simulink model "SimForcesGP2020a"  (R2020b)
settings: Solver=ode4  StartTime=0.0  StopTime=10  FixedStep=0.001  MaxStep=0.001  RelTol=1e-7
values from neighbouring files (symbols this model uses):
  B11_r_B11C = [0.23805608; 0.13201777; 0]    [InitializeSimulationGP.m]
  B11_r_B11Tc1 = [L11; 0; 0]    [InitializeSimulationGP.m]
  B11_Rot_Tc1 = eye(3)    [InitializeSimulationGP.m]
  B11cI = [0.28426000 -0.06487287 0;         -0.06487287  0.54237481 0;                   0  0          0.67891020]    [InitializeSimulationGP.m]
  B12_r_B12C = [0.60504569; 0.27199376; 0.00002484]    [InitializeSimulationGP.m]
  B12_r_B12Tc2 = [L21;0;0]    [InitializeSimulationGP.m]
  B12_Rot_Tc2 = eye(3)    [InitializeSimulationGP.m]
  B12cI = [1.18803886 -2.36786418 0.00280315;          -2.36786418 6.31493281 0.00022322;           0.00280315 0.00022322 7.40915161]    [InitializeSimulationGP.m]
  B31_r_B31C = [0.35781210 0 0]    [InitializeSimulationGP.m]
  B31_Rot_B41 = eye(3)    [InitializeSimulationGP.m]
  B31cI = diag([0.03150902 0.90735702 0.90763033])    [InitializeSimulationGP.m]
  B32_r_B32C = [0.35781210 0 0]    [InitializeSimulationGP.m]
  B32_Rot_B42 = eye(3)    [InitializeSimulationGP.m]
  B32cI = diag([0.03150902 0.90735702 0.90763033])    [InitializeSimulationGP.m]
  B41_r_B41C = [0.55785997 0 0]    [InitializeSimulationGP.m]
  B41_r_B41Tc1 = [lc1;0;0]    [InitializeSimulationGP.m]
  B41cI = diag([0.00370720 0.55759812 0.55785997])    [InitializeSimulationGP.m]
  B42_r_B42C = [0.55785997 0 0]    [InitializeSimulationGP.m]
  B42_r_B42Tc2 = [lc2; 0; 0]    [InitializeSimulationGP.m]
  B42cI = diag([0.00370720 0.55759812 0.55785997])    [InitializeSimulationGP.m]
  B52_r_B52C = [0 0 0.56802906]    [InitializeSimulationGP.m]
  B52_r_B52P32 = [lc3; 0; 0]    [InitializeSimulationGP.m]
  B52_Rot_P32 = eye(3)    [InitializeSimulationGP.m]
  B52cI = diag([0.91789884, 0.91790043, 0.00091463])    [InitializeSimulationGP.m]
  Bc1_r_Bc1B11 = [L1; 0; 0]    [InitializeSimulationGP.m]
  Bc1_r_Bc1B31 = [0;0;0]    [InitializeSimulationGP.m]
  Bc1_r_Bc1C = [0.14178771; 0.16555780; 0]    [InitializeSimulationGP.m]
  Bc1_V = [0;0;0;0;0;0]    [InitializeSimulationGP.m]
  Bc1cI = [+5.892211080 +5.476111360 -0.000019630;          +5.476111360 +28.66965601 -0.000024550;          -0.000019630 -0.000024550 +29.78955950]    [InitializeSimulationGP.m]
  Bc2_r_Bc2B12 = [L2;0;0]    [InitializeSimulationGP.m]
  Bc2_r_Bc2B32 = [0;0;0]    [InitializeSimulationGP.m]
  Bc2_r_Bc2C = [0.54319901; 0.10543875; 0]    [InitializeSimulationGP.m]
  Bc2cI = [0.48071390 0.52924041 0;          0.52924041 5.80912352 0;              0      0          5.97255351]    [InitializeSimulationGP.m]
  beta1 = atan2d(374.261,935)*pi/180    [InitializeSimulationGP.m]
  beta2 = atan2d(45.757,373.313)*pi/180    [InitializeSimulationGP.m]
  beta3 = atan2d(139.50,1132.19)*pi/180    [InitializeSimulationGP.m]
  beta4 = atan2d(88.061,296.198)*pi/180    [InitializeSimulationGP.m]
  D22F = [0;0;0;0;0;0]    [InitializeSimulationGP.m]
  L1 = 1.0071227324212    (= 1.00712273242)    [InitializeSimulationGP.m]
  L11 = 0.37610632101293    (= 0.376106321013)    [InitializeSimulationGP.m]
  L2 = 1.132185817991    (= 1.13218581799)    [InitializeSimulationGP.m]
  L21 = 0.30901132665325    (= 0.309011326653)    [InitializeSimulationGP.m]
  lc1 = 0.745    [InitializeSimulationGP.m]
  lc2 = 0.745    [InitializeSimulationGP.m]
  mB11 = 25.52660174    [InitializeSimulationGP.m]
  mB12 = 33.92850233    [InitializeSimulationGP.m]
  mB31 = 17.36281648    [InitializeSimulationGP.m]
  mB32 = 17.36281648    [InitializeSimulationGP.m]
  mB41 = 10.34519231    [InitializeSimulationGP.m]
  mB42 = 10.34519231    [InitializeSimulationGP.m]
  mB52 = 6.73059863    [InitializeSimulationGP.m]
  mBc1 = 307.29601379    [InitializeSimulationGP.m]
  mBc2 = 54.58702836    [InitializeSimulationGP.m]
  mP22 = 9.26136143    [InitializeSimulationGP.m]
  mP32 = 570.18877059    [InitializeSimulationGP.m]
  P22_r_P22C = [0.62192523 0 0]    [InitializeSimulationGP.m]
  P22_Rot_B52 = eye(3)    [InitializeSimulationGP.m]
  P22cI = diag([0.00662754, 1.48387017, 1.48398069])    [InitializeSimulationGP.m]
  P32_r_P32C = [0.25466704; -0.13034397; -0.01302248]    [InitializeSimulationGP.m]
  P32_r_P32D22 = [0.40499744871392; -0.13130517281345; -0.013385243295654]    [InitializeSimulationGP.m]
  P32_Rot_D22 = [1 0 0;              0 0.9707729441837 0.23999977258512;              0 -0.23999977258512 0.9707729441837]    [InitializeSimulationGP.m]
  P32cI = [46.81220713 0.38607676 -0.00453819;          0.38607676 71.92201786 -1.14320993;          -0.00453819 -1.14320993 67.38128576]    [InitializeSimulationGP.m]
  Tc1_r_Tc1Bc2 = [0.098495302558553; 0.01838181329939; 0]    [InitializeSimulationGP.m]
  Tc1_Rot_Bc2 = [cos(alpha2) -sin(alpha2) 0;                sin(alpha2)  cos(alpha2) 0;                0            0           1]    [InitializeSimulationGP.m]
  Tc2_r_Tc2P22 = [-0.048858374920227;0.36587359346146;0.035276938723102]    [InitializeSimulationGP.m]
  Tc2_Rot_P22 = [0.95853460763586 -0.27664713597974  0.0683942111482;                0.28497614981675  0.93051946315663 -0.23004808784757;                0                 0.23999977258511  0.9707729441837]    [InitializeSimulationGP.m]
  Th1A = 5*pi/180    (= 0.0872664625997)    [InitializeSimulationGP.m]
  Th1B = 20*pi/180    (= 0.349065850399)    [InitializeSimulationGP.m]
  Th1f = 1    [InitializeSimulationGP.m]
  Th2A = 15*pi/180    (= 0.261799387799)    [InitializeSimulationGP.m]
  Th2B = -50*pi/180    (= -0.872664625997)    [InitializeSimulationGP.m]
  Th2f = 2    [InitializeSimulationGP.m]
  W_r_WBc1 = [0.185;-0.085;0]    [InitializeSimulationGP.m]
  W_Rot_Bc1 = [cos(alpha1) -sin(alpha1) 0;              sin(alpha1)  cos(alpha1) 0;              0            0           1]    [InitializeSimulationGP.m]
  Wg = [0; 9.8066; 0]    [InitializeSimulationGP.m]
  x10 = 0.83    [InitializeSimulationGP.m]
  x20 = 0.83    [InitializeSimulationGP.m]
  xf = [1;0;0;0;0;0]    [InitializeSimulationGP.m]
  xt2A = 0.1    [InitializeSimulationGP.m]
  xt2B = 0.5    [InitializeSimulationGP.m]
  xt2f = 1    [InitializeSimulationGP.m]
  ztau = [0;0;0;0;0;1]    [InitializeSimulationGP.m]
undefined symbols (not defined in the file or in its folder): B11_V, B11_V_SS, B11Ftot, B12_U_Tc2, B12_V, B12_V_SS, B12Ftot, B31_r_B31B41, B31_V, B31_V_SS, B31FTot, B32_r_B32B42, B32_U_B42, B32_V, B32_V_SS, B32FTot, B41_V, B41_V_SS, B41FTot, B42_Rot_Tc2, B42_U_Tc2, B42_V, B42_V_SS, B42FTot, B52_U_P32, B52_V, B52_V_SS, B52Ftot, Bc1_V_SS, Bc1Tot, Bc2_Rot_B12, Bc2_Rot_B32, Bc2_U_B12, Bc2_U_B32, Bc2_V, Bc2_V_SS, Bc2Tot, D22_V, D22_V_SS, dq1, dq11, dq12, dq2, dq21, dq22, dx1, dx2, FTot_S1, FTot_S2P, FTot_S2R, P22_r_P22B52, P22_U_B52, P22_V, P22_V_SS, P22FTot, P32_U_D22, P32_V, P32_V_SS, P32FTot, q1 ... (+28)
libraries: nesl_utility x94, sm_lib x45
(part 5 of 6)

== system SimForcesGP2020a/Hydraulic manipulator, calculation/AnalyticVelocities/Structure 2 (Revolute segment)/GeomPropS2R/TiltPistonVelocity ==
  note: Pass to output...
  note: Process data...
  note: Get inputs...
  dq2 : Inport
  x2 : Inport  Port=2
  q2 : Inport  Port=3
  TiltPistonVelocity : MATLAB Function  TreatAsAtomicUnit=on
  dx2 : Outport
  wires:
  dq2/1 -> [dq2]  "dq2"
  [dq2] -> TiltPistonVelocity/3(dq2)  "dq2"
  x2/1 -> [x2]  "x2"
  [x2] -> TiltPistonVelocity/1(x2)  "x2"
  q2/1 -> [q2]  "q2"
  [q2] -> TiltPistonVelocity/2(q2)  "q2"
  [dx2] -> dx2/1  "dx2"
  TiltPistonVelocity/1(dx2) -> [dx2]  "dx2"

== system SimForcesGP2020a/Hydraulic manipulator, calculation/AnalyticVelocities/Structure 2 (Revolute segment)/GeomPropS2R/q21-angle ==
  note: Pass to outputs...
  note: Process data...
  note: Get inputs...
  x2 : Inport
  Fcn : Fcn  Expr=-acos((L21*L21-(u+x20)*(u+x20)-L2*L2)/(-2*(u+x20)*L2))
  q21 : Outport
  wires:
  x2/1 -> [x2]
  [q21] -> q21/1
  [x2] -> Fcn/1
  Fcn/1 -> [q21]

== system SimForcesGP2020a/Hydraulic manipulator, calculation/AnalyticVelocities/Structure 2 (Revolute segment)/GeomPropS2R/q22-angle ==
  note: Get inputs...
  note: Process data...
  note: Pass to outputs...
  x2 : Inport
  Fcn : Fcn  Expr=-acos((L2*L2-(u+x20)*(u+x20)-L21*L21)/(-2*(u+x20)*L21))
  q22 : Outport
  wires:
  [q22] -> q22/1
  Fcn/1 -> [q22]
  [x2] -> Fcn/1
  x2/1 -> [x2]

== system SimForcesGP2020a/Hydraulic manipulator, calculation/AnalyticVelocities/Structure 2 (Revolute segment)/GeomPropS2R/q2Derivative ==
  note: Pass to outputs...
  note: Process data...
  note: Get inputs...
  q2 : Inport
  Derivative4 : Derivative
  dq2 : Outport
  wires:
  q2/1 -> [q2]  "q2"
  [q2] -> Derivative4/1  "q2"
  [dq2] -> dq2/1  "dq2"
  Derivative4/1 -> [dq2]  "dq2"

== matlab function SimForcesGP2020a/Hydraulic manipulator, calculation/AnalyticVelocities/Structure 1/UMatsS1/B41_U_Tc1 ==
  data: B41_r_B41Tc1 input; B41_U_Tc1 output; B41_Rot_Tc1 input
function B41_U_Tc1 = B41_U_Tc1(B41_r_B41Tc1, B41_Rot_Tc1)

B41_U_Tc1 = [B41_Rot_Tc1,                    zeros(3);...
             dual(B41_r_B41Tc1)*B41_Rot_Tc1, B41_Rot_Tc1];
   
end
   
function dual_r = dual(ArAB)

dual_r = [0,  -ArAB(3), ArAB(2);...
          ArAB(3), 0, -ArAB(1);...
          -ArAB(2), ArAB(1), 0];

end

== matlab function SimForcesGP2020a/Hydraulic manipulator, calculation/AnalyticVelocities/Structure 1/RotMatsS1/B41_Rot_Tc1 ==
  data: q12 input; B41_Rot_Tc1 output
function B41_Rot_Tc1 = B41_Rot_Tc1(q12)

B41_Rot_Tc1 = [+cos(q12) -sin(q12) 0;...
               +sin(q12) +cos(q12) 0;...
                   0        0      1];

== matlab function SimForcesGP2020a/Hydraulic manipulator, calculation/AnalyticVelocities/Structure 2 (Prismatic segment)/PosVecsS2P/P22_r_P22B52 ==
  data: xt2 input; P22_r_P22B52 output; P22_r_P22P22p parameter
function P22_r_P22B52 = P22_r_P22B52(xt2, P22_r_P22P22p)

% position vector of {B41} frame at lift piston tip w.r.t. {B31} frame at 
% lift cylinder connection point [m]
P22_r_P22B52 = P22_r_P22P22p + [xt2; 0; 0];

== matlab function SimForcesGP2020a/Hydraulic manipulator, calculation/AnalyticVelocities/Structure 1/UMatsS1/Bc1_U_B11 ==
  data: Bc1_r_Bc1B11 input; Bc1_U_B11 output; Bc1_Rot_B11 input
function Bc1_U_B11 = Bc1_U_B11(Bc1_r_Bc1B11, Bc1_Rot_B11)

Bc1_U_B11 = [Bc1_Rot_B11,                    zeros(3);...
             dual(Bc1_r_Bc1B11)*Bc1_Rot_B11, Bc1_Rot_B11];
   
end
   
function dual_r = dual(ArAB)

dual_r = [0,  -ArAB(3), ArAB(2);...
          ArAB(3), 0, -ArAB(1);...
          -ArAB(2), ArAB(1), 0];

end

== matlab function SimForcesGP2020a/Hydraulic manipulator, calculation/AnalyticVelocities/Structure 2 (Prismatic segment)/UMatsS2P/P22_U_B52 ==
  data: P22_r_P22B52 input; P22_U_B52 output; P22_Rot_B52 input
function P22_U_B52 = P22_U_B52(P22_r_P22B52, P22_Rot_B52)

P22_U_B52 = [P22_Rot_B52,                    zeros(3);...
             dual(P22_r_P22B52)*P22_Rot_B52, P22_Rot_B52];
   
end
   
function dual_r = dual(ArAB)

dual_r = [0,  -ArAB(3), ArAB(2);...
          ArAB(3), 0, -ArAB(1);...
          -ArAB(2), ArAB(1), 0];

end

== matlab function SimForcesGP2020a/Hydraulic manipulator, calculation/AnalyticVelocities/Structure 2 (Prismatic segment)/UMatsS2P/B52_U_P32 ==
  data: B52_r_B52B32 input; B52_U_P32 output; B52_Rot_B32 input
function B52_U_P32 = B52_U_P32(B52_r_B52B32, B52_Rot_B32)

B52_U_P32 = [B52_Rot_B32,                    zeros(3);...
             dual(B52_r_B52B32)*B52_Rot_B32, B52_Rot_B32];
   
end
   
function dual_r = dual(ArAB)

dual_r = [0,  -ArAB(3), ArAB(2);...
          ArAB(3), 0, -ArAB(1);...
          -ArAB(2), ArAB(1), 0];

end

== matlab function SimForcesGP2020a/Hydraulic manipulator, calculation/AnalyticVelocities/Structure 2 (Revolute segment)/PosVecsS2R/B32_r_B32B42 ==
  data: x2 input; B32_r_B32B42 output; B32_r_B32B32p parameter
function B32_r_B32B42 = B32_r_B32B42(x2, B32_r_B32B32p)

B32_r_B32B42 = B32_r_B32B32p + [x2;0;0];

== matlab function SimForcesGP2020a/Hydraulic manipulator, calculation/AnalyticVelocities/Structure 2 (Revolute segment)/RotMatsS2R/B42_Rot_Tc2 ==
  data: q22 input; B42_Rot_Tc2 output
function B42_Rot_Tc2 = B42_Rot_Tc2(q22)

B42_Rot_Tc2 = [+cos(q22) -sin(q22) 0;...
               +sin(q22) +cos(q22) 0;...
                   0        0      1];

== matlab function SimForcesGP2020a/Hydraulic manipulator, calculation/AnalyticVelocities/Structure 2 (Revolute segment)/RotMatsS2R/Bc2_Rot_B12 ==
  data: q2 input; Bc2_Rot_B12 output
function Bc2_Rot_B12 = Bc2_Rot_B12(q2)

Bc2_Rot_B12 = [+cos(q2) -sin(q2) 0;...
               +sin(q2) +cos(q2) 0;...
                  0        0     1];

== matlab function SimForcesGP2020a/Hydraulic manipulator, calculation/AnalyticVelocities/Structure 2 (Revolute segment)/RotMatsS2R/Bc2_Rot_B32 ==
  data: q21 input; Bc2_Rot_B32 output

function Bc2_Rot_B32 = Bc2_Rot_B32(q21)

Bc2_Rot_B32 = [+cos(q21) -sin(q21) 0;...
               +sin(q21) +cos(q21) 0;...
                   0         0     1];

== matlab function SimForcesGP2020a/Hydraulic manipulator, calculation/AnalyticVelocities/Structure 2 (Revolute segment)/UMatS2R/B12_U_Tc2 ==
  data: B12_r_B12Tc2 input; B12_U_Tc2 output; B12_Rot_Tc2 input
function B12_U_Tc2 = B12_U_Tc2(B12_r_B12Tc2, B12_Rot_Tc2)

B12_U_Tc2 = [B12_Rot_Tc2,                    zeros(3);...
             dual(B12_r_B12Tc2)*B12_Rot_Tc2, B12_Rot_Tc2];
   
end
   
function dual_r = dual(ArAB)

dual_r = [0,  -ArAB(3), ArAB(2);...
          ArAB(3), 0, -ArAB(1);...
          -ArAB(2), ArAB(1), 0];

end

== matlab function SimForcesGP2020a/Hydraulic manipulator, calculation/AnalyticVelocities/Structure 2 (Revolute segment)/UMatS2R/B32_U_B42 ==
  data: B32_r_B32B42 input; B32_U_B42 output; B32_Rot_B42 input
function B32_U_B42 = B32_U_B42(B32_r_B32B42, B32_Rot_B42)

B32_U_B42 = [B32_Rot_B42,                    zeros(3);...
             dual(B32_r_B32B42)*B32_Rot_B42, B32_Rot_B42];
   
end
   
function dual_r = dual(ArAB)

dual_r = [0,  -ArAB(3), ArAB(2);...
          ArAB(3), 0, -ArAB(1);...
          -ArAB(2), ArAB(1), 0];

end

== matlab function SimForcesGP2020a/Hydraulic manipulator, calculation/AnalyticVelocities/Structure 2 (Revolute segment)/UMatS2R/B42_U_Tc2 ==
  data: B42_r_B42Tc2 input; B42_U_Tc2 output; B42_Rot_Tc2 input
function B42_U_Tc2 = B42_U_Tc2(B42_r_B42Tc2, B42_Rot_Tc2)

B42_U_Tc2 = [B42_Rot_Tc2,                    zeros(3);...
             dual(B42_r_B42Tc2)*B42_Rot_Tc2, B42_Rot_Tc2];
   
end
   
function dual_r = dual(ArAB)

dual_r = [0,  -ArAB(3), ArAB(2);...
          ArAB(3), 0, -ArAB(1);...
          -ArAB(2), ArAB(1), 0];

end

== matlab function SimForcesGP2020a/Hydraulic manipulator, calculation/AnalyticVelocities/Structure 2 (Revolute segment)/UMatS2R/Bc2_U_B12 ==
  data: Bc2_r_Bc2B12 input; Bc2_U_B12 output; Bc2_Rot_B12 input
function Bc2_U_B12 = Bc2_U_B12(Bc2_r_Bc2B12, Bc2_Rot_B12)

Bc2_U_B12 = [Bc2_Rot_B12,                    zeros(3);...
             dual(Bc2_r_Bc2B12)*Bc2_Rot_B12, Bc2_Rot_B12];
   
end
   
function dual_r = dual(ArAB)

dual_r = [0,  -ArAB(3), ArAB(2);...
          ArAB(3), 0, -ArAB(1);...
          -ArAB(2), ArAB(1), 0];

end

== matlab function SimForcesGP2020a/Hydraulic manipulator, calculation/AnalyticVelocities/Structure 1/RotMatsS1/Bc1_Rot_B11 ==
  data: q1 input; Bc1_Rot_B11 output
function Bc1_Rot_B11 = Bc1_Rot_B11(q1)

Bc1_Rot_B11 = [+cos(q1) -sin(q1) 0;...
               +sin(q1) +cos(q1) 0;...
                  0        0     1];

== matlab function SimForcesGP2020a/Hydraulic manipulator, calculation/AnalyticVelocities/Structure 2 (Revolute segment)/UMatS2R/Bc2_U_B32 ==
  data: Bc2_r_Bc2B32 input; Bc2_U_B32 output; Bc2_Rot_B32 input
function Bc2_U_B32 = Bc2_U_B32(Bc2_r_Bc2B32, Bc2_Rot_B32)

Bc2_U_B32 = [Bc2_Rot_B32,                    zeros(3);...
             dual(Bc2_r_Bc2B32)*Bc2_Rot_B32, Bc2_Rot_B32];
   
end
   
function dual_r = dual(ArAB)

dual_r = [0,  -ArAB(3), ArAB(2);...
          ArAB(3), 0, -ArAB(1);...
          -ArAB(2), ArAB(1), 0];

end

== matlab function SimForcesGP2020a/Hydraulic manipulator, calculation/AnalyticVelocities/Structure 1/UMatsS1/Tc1_U_Bc2 ==
  data: Tc1_r_Tc1Bc2 input; Tc1_U_Bc2 output; Tc1_Rot_Bc2 input
function Tc1_U_Bc2 = Tc1_U_Bc2(Tc1_r_Tc1Bc2, Tc1_Rot_Bc2)

Tc1_U_Bc2 = [Tc1_Rot_Bc2,                    zeros(3);...
             dual(Tc1_r_Tc1Bc2)*Tc1_Rot_Bc2, Tc1_Rot_Bc2];
   
end
   
function dual_r = dual(ArAB)

dual_r = [0,  -ArAB(3), ArAB(2);...
          ArAB(3), 0, -ArAB(1);...
          -ArAB(2), ArAB(1), 0];

end

== matlab function SimForcesGP2020a/Hydraulic manipulator, calculation/AnalyticVelocities/Structure 2 (Revolute segment)/UMatS2R/Tc2_U_P22 ==
  data: Tc2_r_Tc2P22 input; Tc2_U_P22 output; Tc2_Rot_P22 input
function Tc2_U_P22 = Tc2_U_P22(Tc2_r_Tc2P22, Tc2_Rot_P22)

Tc2_U_P22 = [Tc2_Rot_P22,                    zeros(3);...
             dual(Tc2_r_Tc2P22)*Tc2_Rot_P22, Tc2_Rot_P22];
   
end
   
function dual_r = dual(ArAB)

dual_r = [0,  -ArAB(3), ArAB(2);...
          ArAB(3), 0, -ArAB(1);...
          -ArAB(2), ArAB(1), 0];

end

== matlab function SimForcesGP2020a/Hydraulic manipulator, calculation/AnalyticTotalForces/Structure 1/MATLAB Function2 ==
  data: thetaB11 output; B11_r_B11C parameter; mB11 parameter; B11cI parameter
function thetaB11 = thetaB11(B11_r_B11C, mB11, B11cI)

rx = B11_r_B11C(1);
ry = B11_r_B11C(2);
rz = B11_r_B11C(3);

Ixx = B11cI(1,1);
Iyy = B11cI(2,2);
Izz = B11cI(3,3);
Iyz = B11cI(2,3);
Ixz = B11cI(1,3);
Ixy = B11cI(1,2);

t1 = rx*rx;
t2 = ry*ry;
t3 = rz*rz;
t4 = rx*mB11;

thetaB11 = [mB11; rx*mB11; ry*mB11; rz*mB11; t1*mB11; t2*mB11; t3*mB11; t4*ry - Ixy; t4*rz - Ixz; mB11*ry*rz - Iyz; Ixx; Iyy; Izz];

== matlab function SimForcesGP2020a/Hydraulic manipulator, calculation/AnalyticTotalForces/Structure 1/MATLAB Function3 ==
  data: B11V input; B11a input; B11w input; B11dw input; B11_Rot_W input; Wg parameter; YB11 output
function YB11  = thetaBc1(B11V, B11a, B11w, B11dw, B11_Rot_W,  Wg)

vx = B11V(1);
vy = B11V(2);
vz = B11V(3);
ax = B11a(1);
ay = B11a(2);
az = B11a(3);
wx = B11w(1);
wy = B11w(2);
wz = B11w(3);
dwx = B11dw(1);
dwy = B11dw(2);
dwz = B11dw(3);
Bc1g = B11_Rot_W*Wg;
gx = Bc1g(1);
gy = Bc1g(2);
gz = Bc1g(3);

Y11 = ( ax + vz * wy - vy * wz  + gx);
t5 = (wy *  wy);
t6 = (wz * wz);
Y12 = -t5 - t6;
t7 = (wx * wy);
Y13 = (t7 - dwz);
t8 = (wx * wz);
Y14 = (t8 + dwy);
Y15 = 0;
Y16 = 0;
Y17 = 0;
Y18 = 0;
Y19 = 0;
Y110 = 0;
Y111 = 0;
Y112 = 0;
Y113 = 0;
Y21 = vx * wz - vz * wx + ay + gy;
Y22 = t7 + dwz;
t11 = wx * wx;
Y23 = -t11 - t6;
t12 = wy * wz;
Y24 = t12 - dwx;
Y25 = 0;
Y26 = 0;
Y27 = 0;
Y28 = 0;
Y29 = 0;
Y210 = 0;
Y211 = 0;
Y212 = 0;
Y213 = 0;
Y31 = -vx * wy + vy * wx + az + gz;
Y32 = t8 - dwy;
Y33 = t12 + dwx;
Y34 = -t11 - t5;
Y35 = 0;
Y36 = 0;
Y37 = 0;
Y38 = 0;
Y39 = 0;
Y310 = 0;
Y311 = 0;
Y312 = 0;
Y313 = 0;
Y41 = 0;
Y42 = 0;
Y43 = Y31;
Y44 = -Y21;
Y45 = 0;
Y46 = Y33;
Y47 = -Y24;
Y48 = Y32;
Y49 = -Y22;
Y410 = -t5 + t6;
Y411 = dwx;
Y412 = -t12;
Y413 = t12;
Y51 = 0;
Y52 = -Y31;
Y53 = 0;
Y54 = Y11;
Y55 = -Y32;
Y56 = 0;
Y57 = Y14;
Y58 = -Y33;
Y59 = t11 - t6;
Y510 = Y13;
Y511 = t8;
Y512 = dwy;
Y513 = -t8;
Y61 = 0;
Y62 = Y21;
Y63 = -Y11;
Y64 = 0;
Y65 = Y22;
Y66 = -Y13;
Y67 = 0;
Y68 = t5 - t11;
Y69 = Y24;
Y610 = -Y14;
Y611 = -t7;
Y612 = t7;
Y613 = dwz;

YB11 = [Y11 Y12 Y13 Y14 Y15 Y16 Y17 Y18 Y19 Y110 Y111 Y112 Y113;...
        Y21 Y22 Y23 Y24 Y25 Y26 Y27 Y28 Y29 Y210 Y211 Y212 Y213;...
        Y31 Y32 Y33 Y34 Y35 Y36 Y37 Y38 Y39 Y310 Y311 Y312 Y313;...
        Y41 Y42 Y43 Y44 Y45 Y46 Y47 Y48 Y49 Y410 Y411 Y412 Y413;...
        Y51 Y52 Y53 Y54 Y55 Y56 Y57 Y58 Y59 Y510 Y511 Y512 Y513;...
        Y61 Y62 Y63 Y64 Y65 Y66 Y67 Y68 Y69 Y610 Y611 Y612 Y613];

== matlab function SimForcesGP2020a/Hydraulic manipulator, calculation/AnalyticTotalForces/Structure 1/MATLAB Function4 ==
  data: thetaB31 output; B31_r_B31C parameter; mB31 parameter; B31cI parameter
function thetaB31 = thetaB31(B31_r_B31C, mB31, B31cI)

rx = B31_r_B31C(1);
ry = B31_r_B31C(2);
rz = B31_r_B31C(3);

Ixx = B31cI(1,1);
Iyy = B31cI(2,2);
Izz = B31cI(3,3);
Iyz = B31cI(2,3);
Ixz = B31cI(1,3);
Ixy = B31cI(1,2);

t1 = rx*rx;
t2 = ry*ry;
t3 = rz*rz;
t4 = rx*mB31;

thetaB31 = [mB31; rx*mB31; ry*mB31; rz*mB31; t1*mB31; t2*mB31; t3*mB31; t4*ry - Ixy; t4*rz - Ixz; mB31*ry*rz - Iyz; Ixx; Iyy; Izz];

== matlab function SimForcesGP2020a/Hydraulic manipulator, calculation/AnalyticTotalForces/Structure 1/MATLAB Function5 ==
  data: B31V input; B31a input; B31w input; B31dw input; B31_Rot_W input; Wg parameter; YB31 output
function YB31  = thetaBc1(B31V, B31a, B31w, B31dw, B31_Rot_W,  Wg)

vx = B31V(1);
vy = B31V(2);
vz = B31V(3);
ax = B31a(1);
ay = B31a(2);
az = B31a(3);
wx = B31w(1);
wy = B31w(2);
wz = B31w(3);
dwx = B31dw(1);
dwy = B31dw(2);
dwz = B31dw(3);
Bc1g = B31_Rot_W*Wg;
gx = Bc1g(1);
gy = Bc1g(2);
gz = Bc1g(3);

Y11 = ( ax + vz * wy - vy * wz  + gx);
t5 = (wy *  wy);
t6 = (wz * wz);
Y12 = -t5 - t6;
t7 = (wx * wy);
Y13 = (t7 - dwz);
t8 = (wx * wz);
Y14 = (t8 + dwy);
Y15 = 0;
Y16 = 0;
Y17 = 0;
Y18 = 0;
Y19 = 0;
Y110 = 0;
Y111 = 0;
Y112 = 0;
Y113 = 0;
Y21 = vx * wz - vz * wx + ay + gy;
Y22 = t7 + dwz;
t11 = wx * wx;
Y23 = -t11 - t6;
t12 = wy * wz;
Y24 = t12 - dwx;
Y25 = 0;
Y26 = 0;
Y27 = 0;
Y28 = 0;
Y29 = 0;
Y210 = 0;
Y211 = 0;
Y212 = 0;
Y213 = 0;
Y31 = -vx * wy + vy * wx + az + gz;
Y32 = t8 - dwy;
Y33 = t12 + dwx;
Y34 = -t11 - t5;
Y35 = 0;
Y36 = 0;
Y37 = 0;
Y38 = 0;
Y39 = 0;
Y310 = 0;
Y311 = 0;
Y312 = 0;
Y313 = 0;
Y41 = 0;
Y42 = 0;
Y43 = Y31;
Y44 = -Y21;
Y45 = 0;
Y46 = Y33;
Y47 = -Y24;
Y48 = Y32;
Y49 = -Y22;
Y410 = -t5 + t6;
Y411 = dwx;
Y412 = -t12;
Y413 = t12;
Y51 = 0;
Y52 = -Y31;
Y53 = 0;
Y54 = Y11;
Y55 = -Y32;
Y56 = 0;
Y57 = Y14;
Y58 = -Y33;
Y59 = t11 - t6;
Y510 = Y13;
Y511 = t8;
Y512 = dwy;
Y513 = -t8;
Y61 = 0;
Y62 = Y21;
Y63 = -Y11;
Y64 = 0;
Y65 = Y22;
Y66 = -Y13;
Y67 = 0;
Y68 = t5 - t11;
Y69 = Y24;
Y610 = -Y14;
Y611 = -t7;
Y612 = t7;
Y613 = dwz;

YB31 = [Y11 Y12 Y13 Y14 Y15 Y16 Y17 Y18 Y19 Y110 Y111 Y112 Y113;...
        Y21 Y22 Y23 Y24 Y25 Y26 Y27 Y28 Y29 Y210 Y211 Y212 Y213;...
        Y31 Y32 Y33 Y34 Y35 Y36 Y37 Y38 Y39 Y310 Y311 Y312 Y313;...
        Y41 Y42 Y43 Y44 Y45 Y46 Y47 Y48 Y49 Y410 Y411 Y412 Y413;...
        Y51 Y52 Y53 Y54 Y55 Y56 Y57 Y58 Y59 Y510 Y511 Y512 Y513;...
        Y61 Y62 Y63 Y64 Y65 Y66 Y67 Y68 Y69 Y610 Y611 Y612 Y613];

== matlab function SimForcesGP2020a/Hydraulic manipulator, calculation/AnalyticTotalForces/Structure 1/MATLAB Function6 ==
  data: thetaB41 output; B41_r_B41C parameter; mB41 parameter; B41cI parameter
function thetaB41 = thetaB41(B41_r_B41C, mB41, B41cI)

rx = B41_r_B41C(1);
ry = B41_r_B41C(2);
rz = B41_r_B41C(3);

Ixx = B41cI(1,1);
Iyy = B41cI(2,2);
Izz = B41cI(3,3);
Iyz = B41cI(2,3);
Ixz = B41cI(1,3);
Ixy = B41cI(1,2);

t1 = rx*rx;
t2 = ry*ry;
t3 = rz*rz;
t4 = rx*mB41;

thetaB41 = [mB41; rx*mB41; ry*mB41; rz*mB41; t1*mB41; t2*mB41; t3*mB41; t4*ry - Ixy; t4*rz - Ixz; mB41*ry*rz - Iyz; Ixx; Iyy; Izz];

== matlab function SimForcesGP2020a/Hydraulic manipulator, calculation/AnalyticVelocities/Structure 1/UMatsS1/B11_U_Tc1 ==
  data: B11_r_B11Tc1 input; B11_U_Tc1 output; B11_Rot_Tc1 input
function B11_U_Tc1 = B11_U_Tc1(B11_r_B11Tc1, B11_Rot_Tc1)

B11_U_Tc1 = [B11_Rot_Tc1,                    zeros(3);...
             dual(B11_r_B11Tc1)*B11_Rot_Tc1, B11_Rot_Tc1];
   
end
   
function dual_r = dual(ArAB)

dual_r = [0,  -ArAB(3), ArAB(2);...
          ArAB(3), 0, -ArAB(1);...
          -ArAB(2), ArAB(1), 0];

end

== matlab function SimForcesGP2020a/Hydraulic manipulator, calculation/AnalyticTotalForces/Structure 1/MATLAB Function7 ==
  data: B41V input; B41a input; B41w input; B41dw input; B41_Rot_W input; Wg parameter; YB41 output
function YB41  = thetaB41(B41V, B41a, B41w, B41dw, B41_Rot_W,  Wg)

vx = B41V(1);
vy = B41V(2);
vz = B41V(3);
ax = B41a(1);
ay = B41a(2);
az = B41a(3);
wx = B41w(1);
wy = B41w(2);
wz = B41w(3);
dwx = B41dw(1);
dwy = B41dw(2);
dwz = B41dw(3);
Bc1g = B41_Rot_W*Wg;
gx = Bc1g(1);
gy = Bc1g(2);
gz = Bc1g(3);

Y11 = ( ax + vz * wy - vy * wz  + gx);
t5 = (wy *  wy);
t6 = (wz * wz);
Y12 = -t5 - t6;
t7 = (wx * wy);
Y13 = (t7 - dwz);
t8 = (wx * wz);
Y14 = (t8 + dwy);
Y15 = 0;
Y16 = 0;
Y17 = 0;
Y18 = 0;
Y19 = 0;
Y110 = 0;
Y111 = 0;
Y112 = 0;
Y113 = 0;
Y21 = vx * wz - vz * wx + ay + gy;
Y22 = t7 + dwz;
t11 = wx * wx;
Y23 = -t11 - t6;
t12 = wy * wz;
Y24 = t12 - dwx;
Y25 = 0;
Y26 = 0;
Y27 = 0;
Y28 = 0;
Y29 = 0;
Y210 = 0;
Y211 = 0;
Y212 = 0;
Y213 = 0;
Y31 = -vx * wy + vy * wx + az + gz;
Y32 = t8 - dwy;
Y33 = t12 + dwx;
Y34 = -t11 - t5;
Y35 = 0;
Y36 = 0;
Y37 = 0;
Y38 = 0;
Y39 = 0;
Y310 = 0;
Y311 = 0;
Y312 = 0;
Y313 = 0;
Y41 = 0;
Y42 = 0;
Y43 = Y31;
Y44 = -Y21;
Y45 = 0;
Y46 = Y33;
Y47 = -Y24;
Y48 = Y32;
Y49 = -Y22;
Y410 = -t5 + t6;
Y411 = dwx;
Y412 = -t12;
Y413 = t12;
Y51 = 0;
Y52 = -Y31;
Y53 = 0;
Y54 = Y11;
Y55 = -Y32;
Y56 = 0;
Y57 = Y14;
Y58 = -Y33;
Y59 = t11 - t6;
Y510 = Y13;
Y511 = t8;
Y512 = dwy;
Y513 = -t8;
Y61 = 0;
Y62 = Y21;
Y63 = -Y11;
Y64 = 0;
Y65 = Y22;
Y66 = -Y13;
Y67 = 0;
Y68 = t5 - t11;
Y69 = Y24;
Y610 = -Y14;
Y611 = -t7;
Y612 = t7;
Y613 = dwz;

YB41 = [Y11 Y12 Y13 Y14 Y15 Y16 Y17 Y18 Y19 Y110 Y111 Y112 Y113;...
        Y21 Y22 Y23 Y24 Y25 Y26 Y27 Y28 Y29 Y210 Y211 Y212 Y213;...
        Y31 Y32 Y33 Y34 Y35 Y36 Y37 Y38 Y39 Y310 Y311 Y312 Y313;...
        Y41 Y42 Y43 Y44 Y45 Y46 Y47 Y48 Y49 Y410 Y411 Y412 Y413;...
        Y51 Y52 Y53 Y54 Y55 Y56 Y57 Y58 Y59 Y510 Y511 Y512 Y513;...
        Y61 Y62 Y63 Y64 Y65 Y66 Y67 Y68 Y69 Y610 Y611 Y612 Y613];

== matlab function SimForcesGP2020a/Hydraulic manipulator, calculation/AnalyticTotalForces/Structure 2 (Revolute segment)/MATLAB Function2 ==
  data: thetaB12 output; B12_r_B12C parameter; mB12 parameter; B12cI parameter
function thetaB12 = thetaB12(B12_r_B12C, mB12, B12cI)

rx = B12_r_B12C(1);
ry = B12_r_B12C(2);
rz = B12_r_B12C(3);

Ixx = B12cI(1,1);
Iyy = B12cI(2,2);
Izz = B12cI(3,3);
Iyz = B12cI(2,3);
Ixz = B12cI(1,3);
Ixy = B12cI(1,2);

t1 = rx*rx;
t2 = ry*ry;
t3 = rz*rz;
t4 = rx*mB12;

thetaB12 = [mB12; rx*mB12; ry*mB12; rz*mB12; t1*mB12; t2*mB12; t3*mB12; t4*ry - Ixy; t4*rz - Ixz; mB12*ry*rz - Iyz; Ixx; Iyy; Izz];

== matlab function SimForcesGP2020a/Hydraulic manipulator, calculation/AnalyticTotalForces/Structure 2 (Revolute segment)/MATLAB Function4 ==
  data: thetaB32 output; B32_r_B32C parameter; mB32 parameter; B32cI parameter
function thetaB32 = thetaB32(B32_r_B32C, mB32, B32cI)

rx = B32_r_B32C(1);
ry = B32_r_B32C(2);
rz = B32_r_B32C(3);

Ixx = B32cI(1,1);
Iyy = B32cI(2,2);
Izz = B32cI(3,3);
Iyz = B32cI(2,3);
Ixz = B32cI(1,3);
Ixy = B32cI(1,2);

t1 = rx*rx;
t2 = ry*ry;
t3 = rz*rz;
t4 = rx*mB32;

thetaB32 = [mB32; rx*mB32; ry*mB32; rz*mB32; t1*mB32; t2*mB32; t3*mB32; t4*ry - Ixy; t4*rz - Ixz; mB32*ry*rz - Iyz; Ixx; Iyy; Izz];

== matlab function SimForcesGP2020a/Hydraulic manipulator, calculation/AnalyticTotalForces/Structure 2 (Revolute segment)/MATLAB Function6 ==
  data: thetaB42 output; B42_r_B42C parameter; mB42 parameter; B42cI parameter
function thetaB42 = thetaB42(B42_r_B42C, mB42, B42cI)

rx = B42_r_B42C(1);
ry = B42_r_B42C(2);
rz = B42_r_B42C(3);

Ixx = B42cI(1,1);
Iyy = B42cI(2,2);
Izz = B42cI(3,3);
Iyz = B42cI(2,3);
Ixz = B42cI(1,3);
Ixy = B42cI(1,2);

t1 = rx*rx;
t2 = ry*ry;
t3 = rz*rz;
t4 = rx*mB42;

thetaB42 = [mB42; rx*mB42; ry*mB42; rz*mB42; t1*mB42; t2*mB42; t3*mB42; t4*ry - Ixy; t4*rz - Ixz; mB42*ry*rz - Iyz; Ixx; Iyy; Izz];

== matlab function SimForcesGP2020a/Hydraulic manipulator, calculation/AnalyticTotalForces/Structure 2 (Revolute segment)/MATLAB Function ==
  data: thetaBc2 output; Bc2_r_Bc2C parameter; mBc2 parameter; Bc2cI parameter
function thetaBc2 = thetaBc2(Bc2_r_Bc2C, mBc2, Bc2cI)

rx = Bc2_r_Bc2C(1);
ry = Bc2_r_Bc2C(2);
rz = Bc2_r_Bc2C(3);

Ixx = Bc2cI(1,1);
Iyy = Bc2cI(2,2);
Izz = Bc2cI(3,3);
Iyz = Bc2cI(2,3);
Ixz = Bc2cI(1,3);
Ixy = Bc2cI(1,2);

t1 = rx*rx;
t2 = ry*ry;
t3 = rz*rz;
t4 = rx*mBc2;

thetaBc2 = [mBc2; rx*mBc2; ry*mBc2; rz*mBc2; t1*mBc2; t2*mBc2; t3*mBc2; t4*ry - Ixy; t4*rz - Ixz; mBc2*ry*rz - Iyz; Ixx; Iyy; Izz];

== matlab function SimForcesGP2020a/Hydraulic manipulator, calculation/AnalyticTotalForces/Structure 2 (Revolute segment)/MATLAB Function3 ==
  data: B12V input; B12a input; B12w input; B12dw input; B12_Rot_W input; Wg parameter; YB12 output
function YB12  = thetaB12(B12V, B12a, B12w, B12dw, B12_Rot_W,  Wg)

vx = B12V(1);
vy = B12V(2);
vz = B12V(3);
ax = B12a(1);
ay = B12a(2);
az = B12a(3);
wx = B12w(1);
wy = B12w(2);
wz = B12w(3);
dwx = B12dw(1);
dwy = B12dw(2);
dwz = B12dw(3);
B12g = B12_Rot_W*Wg;
gx = B12g(1);
gy = B12g(2);
gz = B12g(3);

Y11 = ( ax + vz * wy - vy * wz  + gx);
t5 = (wy *  wy);
t6 = (wz * wz);
Y12 = -t5 - t6;
t7 = (wx * wy);
Y13 = (t7 - dwz);
t8 = (wx * wz);
Y14 = (t8 + dwy);
Y15 = 0;
Y16 = 0;
Y17 = 0;
Y18 = 0;
Y19 = 0;
Y110 = 0;
Y111 = 0;
Y112 = 0;
Y113 = 0;
Y21 = vx * wz - vz * wx + ay + gy;
Y22 = t7 + dwz;
t11 = wx * wx;
Y23 = -t11 - t6;
t12 = wy * wz;
Y24 = t12 - dwx;
Y25 = 0;
Y26 = 0;
Y27 = 0;
Y28 = 0;
Y29 = 0;
Y210 = 0;
Y211 = 0;
Y212 = 0;
Y213 = 0;
Y31 = -vx * wy + vy * wx + az + gz;
Y32 = t8 - dwy;
Y33 = t12 + dwx;
Y34 = -t11 - t5;
Y35 = 0;
Y36 = 0;
Y37 = 0;
Y38 = 0;
Y39 = 0;
Y310 = 0;
Y311 = 0;
Y312 = 0;
Y313 = 0;
Y41 = 0;
Y42 = 0;
Y43 = Y31;
Y44 = -Y21;
Y45 = 0;
Y46 = Y33;
Y47 = -Y24;
Y48 = Y32;
Y49 = -Y22;
Y410 = -t5 + t6;
Y411 = dwx;
Y412 = -t12;
Y413 = t12;
Y51 = 0;
Y52 = -Y31;
Y53 = 0;
Y54 = Y11;
Y55 = -Y32;
Y56 = 0;
Y57 = Y14;
Y58 = -Y33;
Y59 = t11 - t6;
Y510 = Y13;
Y511 = t8;
Y512 = dwy;
Y513 = -t8;
Y61 = 0;
Y62 = Y21;
Y63 = -Y11;
Y64 = 0;
Y65 = Y22;
Y66 = -Y13;
Y67 = 0;
Y68 = t5 - t11;
Y69 = Y24;
Y610 = -Y14;
Y611 = -t7;
Y612 = t7;
Y613 = dwz;

YB12 = [Y11 Y12 Y13 Y14 Y15 Y16 Y17 Y18 Y19 Y110 Y111 Y112 Y113;...
        Y21 Y22 Y23 Y24 Y25 Y26 Y27 Y28 Y29 Y210 Y211 Y212 Y213;...
        Y31 Y32 Y33 Y34 Y35 Y36 Y37 Y38 Y39 Y310 Y311 Y312 Y313;...
        Y41 Y42 Y43 Y44 Y45 Y46 Y47 Y48 Y49 Y410 Y411 Y412 Y413;...
        Y51 Y52 Y53 Y54 Y55 Y56 Y57 Y58 Y59 Y510 Y511 Y512 Y513;...
        Y61 Y62 Y63 Y64 Y65 Y66 Y67 Y68 Y69 Y610 Y611 Y612 Y613];

== matlab function SimForcesGP2020a/Hydraulic manipulator, calculation/AnalyticTotalForces/Structure 2 (Revolute segment)/MATLAB Function5 ==
  data: B32V input; B32a input; B32w input; B32dw input; B32_Rot_W input; Wg parameter; YB32 output
function YB32  = thetaB32(B32V, B32a, B32w, B32dw, B32_Rot_W,  Wg)

vx = B32V(1);
vy = B32V(2);
vz = B32V(3);
ax = B32a(1);
ay = B32a(2);
az = B32a(3);
wx = B32w(1);
wy = B32w(2);
wz = B32w(3);
dwx = B32dw(1);
dwy = B32dw(2);
dwz = B32dw(3);
B32g = B32_Rot_W*Wg;
gx = B32g(1);
gy = B32g(2);
gz = B32g(3);

Y11 = ( ax + vz * wy - vy * wz  + gx);
t5 = (wy *  wy);
t6 = (wz * wz);
Y12 = -t5 - t6;
t7 = (wx * wy);
Y13 = (t7 - dwz);
t8 = (wx * wz);
Y14 = (t8 + dwy);
Y15 = 0;
Y16 = 0;
Y17 = 0;
Y18 = 0;
Y19 = 0;
Y110 = 0;
Y111 = 0;
Y112 = 0;
Y113 = 0;
Y21 = vx * wz - vz * wx + ay + gy;
Y22 = t7 + dwz;
t11 = wx * wx;
Y23 = -t11 - t6;
t12 = wy * wz;
Y24 = t12 - dwx;
Y25 = 0;
Y26 = 0;
Y27 = 0;
Y28 = 0;
Y29 = 0;
Y210 = 0;
Y211 = 0;
Y212 = 0;
Y213 = 0;
Y31 = -vx * wy + vy * wx + az + gz;
Y32 = t8 - dwy;
Y33 = t12 + dwx;
Y34 = -t11 - t5;
Y35 = 0;
Y36 = 0;
Y37 = 0;
Y38 = 0;
Y39 = 0;
Y310 = 0;
Y311 = 0;
Y312 = 0;
Y313 = 0;
Y41 = 0;
Y42 = 0;
Y43 = Y31;
Y44 = -Y21;
Y45 = 0;
Y46 = Y33;
Y47 = -Y24;
Y48 = Y32;
Y49 = -Y22;
Y410 = -t5 + t6;
Y411 = dwx;
Y412 = -t12;
Y413 = t12;
Y51 = 0;
Y52 = -Y31;
Y53 = 0;
Y54 = Y11;
Y55 = -Y32;
Y56 = 0;
Y57 = Y14;
Y58 = -Y33;
Y59 = t11 - t6;
Y510 = Y13;
Y511 = t8;
Y512 = dwy;
Y513 = -t8;
Y61 = 0;
Y62 = Y21;
Y63 = -Y11;
Y64 = 0;
Y65 = Y22;
Y66 = -Y13;
Y67 = 0;
Y68 = t5 - t11;
Y69 = Y24;
Y610 = -Y14;
Y611 = -t7;
Y612 = t7;
Y613 = dwz;

YB32 = [Y11 Y12 Y13 Y14 Y15 Y16 Y17 Y18 Y19 Y110 Y111 Y112 Y113;...
        Y21 Y22 Y23 Y24 Y25 Y26 Y27 Y28 Y29 Y210 Y211 Y212 Y213;...
        Y31 Y32 Y33 Y34 Y35 Y36 Y37 Y38 Y39 Y310 Y311 Y312 Y313;...
        Y41 Y42 Y43 Y44 Y45 Y46 Y47 Y48 Y49 Y410 Y411 Y412 Y413;...
        Y51 Y52 Y53 Y54 Y55 Y56 Y57 Y58 Y59 Y510 Y511 Y512 Y513;...
        Y61 Y62 Y63 Y64 Y65 Y66 Y67 Y68 Y69 Y610 Y611 Y612 Y613];

== matlab function SimForcesGP2020a/Hydraulic manipulator, calculation/AnalyticTotalForces/Structure 2 (Revolute segment)/MATLAB Function7 ==
  data: B42V input; B42a input; B42w input; B42dw input; B42_Rot_W input; Wg parameter; YB42 output
function YB42  = thetaB42(B42V, B42a, B42w, B42dw, B42_Rot_W,  Wg)

vx = B42V(1);
vy = B42V(2);
vz = B42V(3);
ax = B42a(1);
ay = B42a(2);
az = B42a(3);
wx = B42w(1);
wy = B42w(2);
wz = B42w(3);
dwx = B42dw(1);
dwy = B42dw(2);
dwz = B42dw(3);
B42g = B42_Rot_W*Wg;
gx = B42g(1);
gy = B42g(2);
gz = B42g(3);

Y11 = ( ax + vz * wy - vy * wz  + gx);
t5 = (wy *  wy);
t6 = (wz * wz);
Y12 = -t5 - t6;
t7 = (wx * wy);
Y13 = (t7 - dwz);
t8 = (wx * wz);
Y14 = (t8 + dwy);
Y15 = 0;
Y16 = 0;
Y17 = 0;
Y18 = 0;
Y19 = 0;
Y110 = 0;
Y111 = 0;
Y112 = 0;
Y113 = 0;
Y21 = vx * wz - vz * wx + ay + gy;
Y22 = t7 + dwz;
t11 = wx * wx;
Y23 = -t11 - t6;
t12 = wy * wz;
Y24 = t12 - dwx;
Y25 = 0;
Y26 = 0;
Y27 = 0;
Y28 = 0;
Y29 = 0;
Y210 = 0;
Y211 = 0;
Y212 = 0;
Y213 = 0;
Y31 = -vx * wy + vy * wx + az + gz;
Y32 = t8 - dwy;
Y33 = t12 + dwx;
Y34 = -t11 - t5;
Y35 = 0;
Y36 = 0;
Y37 = 0;
Y38 = 0;
Y39 = 0;
Y310 = 0;
Y311 = 0;
Y312 = 0;
Y313 = 0;
Y41 = 0;
Y42 = 0;
Y43 = Y31;
Y44 = -Y21;
Y45 = 0;
Y46 = Y33;
Y47 = -Y24;
Y48 = Y32;
Y49 = -Y22;
Y410 = -t5 + t6;
Y411 = dwx;
Y412 = -t12;
Y413 = t12;
Y51 = 0;
Y52 = -Y31;
Y53 = 0;
Y54 = Y11;
Y55 = -Y32;
Y56 = 0;
Y57 = Y14;
Y58 = -Y33;
Y59 = t11 - t6;
Y510 = Y13;
Y511 = t8;
Y512 = dwy;
Y513 = -t8;
Y61 = 0;
Y62 = Y21;
Y63 = -Y11;
Y64 = 0;
Y65 = Y22;
Y66 = -Y13;
Y67 = 0;
Y68 = t5 - t11;
Y69 = Y24;
Y610 = -Y14;
Y611 = -t7;
Y612 = t7;
Y613 = dwz;

YB42 = [Y11 Y12 Y13 Y14 Y15 Y16 Y17 Y18 Y19 Y110 Y111 Y112 Y113;...
        Y21 Y22 Y23 Y24 Y25 Y26 Y27 Y28 Y29 Y210 Y211 Y212 Y213;...
        Y31 Y32 Y33 Y34 Y35 Y36 Y37 Y38 Y39 Y310 Y311 Y312 Y313;...
        Y41 Y42 Y43 Y44 Y45 Y46 Y47 Y48 Y49 Y410 Y411 Y412 Y413;...
        Y51 Y52 Y53 Y54 Y55 Y56 Y57 Y58 Y59 Y510 Y511 Y512 Y513;...
        Y61 Y62 Y63 Y64 Y65 Y66 Y67 Y68 Y69 Y610 Y611 Y612 Y613];

== matlab function SimForcesGP2020a/Hydraulic manipulator, calculation/AnalyticVelocities/Structure 1/GeomPropS1/Subsystem/LiftPistonVelocity ==
  data: dq1 input; x1 input; q1 input; dx1 output; L1 parameter; L11 parameter; x10 parameter
function dx1 = dx1(dq1, x1, q1, L1, L11, x10)

dx1 = -(L1*L11*sin(q1))/(x1+x10)*dq1;

== matlab function SimForcesGP2020a/Hydraulic manipulator, calculation/AnalyticTotalForces/Structure 2 (Revolute segment)/MATLAB Function1 ==
  data: Bc2V input; Bc2a input; Bc2w input; Bc2dw input; Bc2_Rot_W input; Wg parameter; YBc2 output
function YBc2  = thetaBc2(Bc2V, Bc2a, Bc2w, Bc2dw, Bc2_Rot_W,  Wg)

vx = Bc2V(1);
vy = Bc2V(2);
vz = Bc2V(3);
ax = Bc2a(1);
ay = Bc2a(2);
az = Bc2a(3);
wx = Bc2w(1);
wy = Bc2w(2);
wz = Bc2w(3);
dwx = Bc2dw(1);
dwy = Bc2dw(2);
dwz = Bc2dw(3);
Bc2g = Bc2_Rot_W*Wg;
gx = Bc2g(1);
gy = Bc2g(2);
gz = Bc2g(3);

Y11 = ( ax + vz * wy - vy * wz  + gx);
t5 = (wy *  wy);
t6 = (wz * wz);
Y12 = -t5 - t6;
t7 = (wx * wy);
Y13 = (t7 - dwz);
t8 = (wx * wz);
Y14 = (t8 + dwy);
Y15 = 0;
Y16 = 0;
Y17 = 0;
Y18 = 0;
Y19 = 0;
Y110 = 0;
Y111 = 0;
Y112 = 0;
Y113 = 0;
Y21 = vx * wz - vz * wx + ay + gy;
Y22 = t7 + dwz;
t11 = wx * wx;
Y23 = -t11 - t6;
t12 = wy * wz;
Y24 = t12 - dwx;
Y25 = 0;
Y26 = 0;
Y27 = 0;
Y28 = 0;
Y29 = 0;
Y210 = 0;
Y211 = 0;
Y212 = 0;
Y213 = 0;
Y31 = -vx * wy + vy * wx + az + gz;
Y32 = t8 - dwy;
Y33 = t12 + dwx;
Y34 = -t11 - t5;
Y35 = 0;
Y36 = 0;
Y37 = 0;
Y38 = 0;
Y39 = 0;
Y310 = 0;
Y311 = 0;
Y312 = 0;
Y313 = 0;
Y41 = 0;
Y42 = 0;
Y43 = Y31;
Y44 = -Y21;
Y45 = 0;
Y46 = Y33;
Y47 = -Y24;
Y48 = Y32;
Y49 = -Y22;
Y410 = -t5 + t6;
Y411 = dwx;
Y412 = -t12;
Y413 = t12;
Y51 = 0;
Y52 = -Y31;
Y53 = 0;
Y54 = Y11;
Y55 = -Y32;
Y56 = 0;
Y57 = Y14;
Y58 = -Y33;
Y59 = t11 - t6;
Y510 = Y13;
Y511 = t8;
Y512 = dwy;
Y513 = -t8;
Y61 = 0;
Y62 = Y21;
Y63 = -Y11;
Y64 = 0;
Y65 = Y22;
Y66 = -Y13;
Y67 = 0;
Y68 = t5 - t11;
Y69 = Y24;
Y610 = -Y14;
Y611 = -t7;
Y612 = t7;
Y613 = dwz;

YBc2 = [Y11 Y12 Y13 Y14 Y15 Y16 Y17 Y18 Y19 Y110 Y111 Y112 Y113;...
        Y21 Y22 Y23 Y24 Y25 Y26 Y27 Y28 Y29 Y210 Y211 Y212 Y213;...
        Y31 Y32 Y33 Y34 Y35 Y36 Y37 Y38 Y39 Y310 Y311 Y312 Y313;...
        Y41 Y42 Y43 Y44 Y45 Y46 Y47 Y48 Y49 Y410 Y411 Y412 Y413;...
        Y51 Y52 Y53 Y54 Y55 Y56 Y57 Y58 Y59 Y510 Y511 Y512 Y513;...
        Y61 Y62 Y63 Y64 Y65 Y66 Y67 Y68 Y69 Y610 Y611 Y612 Y613];

== matlab function SimForcesGP2020a/Hydraulic manipulator, calculation/AnalyticTotalForces/Structure 2 (Prismatic segment)/MATLAB Function6 ==
  data: thetaP22 output; P22_r_P22C parameter; mP22 parameter; P22cI parameter
function thetaP22 = thetaP22(P22_r_P22C, mP22, P22cI)

rx = P22_r_P22C(1);
ry = P22_r_P22C(2);
rz = P22_r_P22C(3);

Ixx = P22cI(1,1);
Iyy = P22cI(2,2);
Izz = P22cI(3,3);
Iyz = P22cI(2,3);
Ixz = P22cI(1,3);
Ixy = P22cI(1,2);

t1 = rx*rx;
t2 = ry*ry;
t3 = rz*rz;
t4 = rx*mP22;

thetaP22 = [mP22; rx*mP22; ry*mP22; rz*mP22; t1*mP22; t2*mP22; t3*mP22; t4*ry - Ixy; t4*rz - Ixz; mP22*ry*rz - Iyz; Ixx; Iyy; Izz];

== matlab function SimForcesGP2020a/Hydraulic manipulator, calculation/AnalyticTotalForces/Structure 2 (Prismatic segment)/MATLAB Function7 ==
  data: P22V input; P22a input; P22w input; P22dw input; P22_Rot_W input; Wg parameter; YP22 output
function YP22  = thetaP22(P22V, P22a, P22w, P22dw, P22_Rot_W,  Wg)

vx = P22V(1);
vy = P22V(2);
vz = P22V(3);
ax = P22a(1);
ay = P22a(2);
az = P22a(3);
wx = P22w(1);
wy = P22w(2);
wz = P22w(3);
dwx = P22dw(1);
dwy = P22dw(2);
dwz = P22dw(3);
P22g = P22_Rot_W*Wg;
gx = P22g(1);
gy = P22g(2);
gz = P22g(3);

Y11 = ( ax + vz * wy - vy * wz  + gx);
t5 = (wy *  wy);
t6 = (wz * wz);
Y12 = -t5 - t6;
t7 = (wx * wy);
Y13 = (t7 - dwz);
t8 = (wx * wz);
Y14 = (t8 + dwy);
Y15 = 0;
Y16 = 0;
Y17 = 0;
Y18 = 0;
Y19 = 0;
Y110 = 0;
Y111 = 0;
Y112 = 0;
Y113 = 0;
Y21 = vx * wz - vz * wx + ay + gy;
Y22 = t7 + dwz;
t11 = wx * wx;
Y23 = -t11 - t6;
t12 = wy * wz;
Y24 = t12 - dwx;
Y25 = 0;
Y26 = 0;
Y27 = 0;
Y28 = 0;
Y29 = 0;
Y210 = 0;
Y211 = 0;
Y212 = 0;
Y213 = 0;
Y31 = -vx * wy + vy * wx + az + gz;
Y32 = t8 - dwy;
Y33 = t12 + dwx;
Y34 = -t11 - t5;
Y35 = 0;
Y36 = 0;
Y37 = 0;
Y38 = 0;
Y39 = 0;
Y310 = 0;
Y311 = 0;
Y312 = 0;
Y313 = 0;
Y41 = 0;
Y42 = 0;
Y43 = Y31;
Y44 = -Y21;
Y45 = 0;
Y46 = Y33;
Y47 = -Y24;
Y48 = Y32;
Y49 = -Y22;
Y410 = -t5 + t6;
Y411 = dwx;
Y412 = -t12;
Y413 = t12;
Y51 = 0;
Y52 = -Y31;
Y53 = 0;
Y54 = Y11;
Y55 = -Y32;
Y56 = 0;
Y57 = Y14;
Y58 = -Y33;
Y59 = t11 - t6;
Y510 = Y13;
Y511 = t8;
Y512 = dwy;
Y513 = -t8;
Y61 = 0;
Y62 = Y21;
Y63 = -Y11;
Y64 = 0;
Y65 = Y22;
Y66 = -Y13;
Y67 = 0;
Y68 = t5 - t11;
Y69 = Y24;
Y610 = -Y14;
Y611 = -t7;
Y612 = t7;
Y613 = dwz;

YP22 = [Y11 Y12 Y13 Y14 Y15 Y16 Y17 Y18 Y19 Y110 Y111 Y112 Y113;...
        Y21 Y22 Y23 Y24 Y25 Y26 Y27 Y28 Y29 Y210 Y211 Y212 Y213;...
        Y31 Y32 Y33 Y34 Y35 Y36 Y37 Y38 Y39 Y310 Y311 Y312 Y313;...
        Y41 Y42 Y43 Y44 Y45 Y46 Y47 Y48 Y49 Y410 Y411 Y412 Y413;...
        Y51 Y52 Y53 Y54 Y55 Y56 Y57 Y58 Y59 Y510 Y511 Y512 Y513;...
        Y61 Y62 Y63 Y64 Y65 Y66 Y67 Y68 Y69 Y610 Y611 Y612 Y613];

== matlab function SimForcesGP2020a/Hydraulic manipulator, calculation/AnalyticTotalForces/Structure 2 (Prismatic segment)/MATLAB Function1 ==
  data: thetaB52 output; B52_r_B52C parameter; mB52 parameter; B52cI parameter
function thetaB52 = thetaB52(B52_r_B52C, mB52, B52cI)

rx = B52_r_B52C(1);
ry = B52_r_B52C(2);
rz = B52_r_B52C(3);

Ixx = B52cI(1,1);
Iyy = B52cI(2,2);
Izz = B52cI(3,3);
Iyz = B52cI(2,3);
Ixz = B52cI(1,3);
Ixy = B52cI(1,2);

t1 = rx*rx;
t2 = ry*ry;
t3 = rz*rz;
t4 = rx*mB52;

thetaB52 = [mB52; rx*mB52; ry*mB52; rz*mB52; t1*mB52; t2*mB52; t3*mB52; t4*ry - Ixy; t4*rz - Ixz; mB52*ry*rz - Iyz; Ixx; Iyy; Izz];

== matlab function SimForcesGP2020a/Hydraulic manipulator, calculation/AnalyticTotalForces/Structure 2 (Prismatic segment)/MATLAB Function2 ==
  data: B52V input; B52a input; B52w input; B52dw input; B52_Rot_W input; Wg parameter; YB52 output
function YB52  = thetaB52(B52V, B52a, B52w, B52dw, B52_Rot_W,  Wg)

vx = B52V(1);
vy = B52V(2);
vz = B52V(3);
ax = B52a(1);
ay = B52a(2);
az = B52a(3);
wx = B52w(1);
wy = B52w(2);
wz = B52w(3);
dwx = B52dw(1);
dwy = B52dw(2);
dwz = B52dw(3);
B52g = B52_Rot_W*Wg;
gx = B52g(1);
gy = B52g(2);
gz = B52g(3);

Y11 = ( ax + vz * wy - vy * wz  + gx);
t5 = (wy *  wy);
t6 = (wz * wz);
Y12 = -t5 - t6;
t7 = (wx * wy);
Y13 = (t7 - dwz);
t8 = (wx * wz);
Y14 = (t8 + dwy);
Y15 = 0;
Y16 = 0;
Y17 = 0;
Y18 = 0;
Y19 = 0;
Y110 = 0;
Y111 = 0;
Y112 = 0;
Y113 = 0;
Y21 = vx * wz - vz * wx + ay + gy;
Y22 = t7 + dwz;
t11 = wx * wx;
Y23 = -t11 - t6;
t12 = wy * wz;
Y24 = t12 - dwx;
Y25 = 0;
Y26 = 0;
Y27 = 0;
Y28 = 0;
Y29 = 0;
Y210 = 0;
Y211 = 0;
Y212 = 0;
Y213 = 0;
Y31 = -vx * wy + vy * wx + az + gz;
Y32 = t8 - dwy;
Y33 = t12 + dwx;
Y34 = -t11 - t5;
Y35 = 0;
Y36 = 0;
Y37 = 0;
Y38 = 0;
Y39 = 0;
Y310 = 0;
Y311 = 0;
Y312 = 0;
Y313 = 0;
Y41 = 0;
Y42 = 0;
Y43 = Y31;
Y44 = -Y21;
Y45 = 0;
Y46 = Y33;
Y47 = -Y24;
Y48 = Y32;
Y49 = -Y22;
Y410 = -t5 + t6;
Y411 = dwx;
Y412 = -t12;
Y413 = t12;
Y51 = 0;
Y52 = -Y31;
Y53 = 0;
Y54 = Y11;
Y55 = -Y32;
Y56 = 0;
Y57 = Y14;
Y58 = -Y33;
Y59 = t11 - t6;
Y510 = Y13;
Y511 = t8;
Y512 = dwy;
Y513 = -t8;
Y61 = 0;
Y62 = Y21;
Y63 = -Y11;
Y64 = 0;
Y65 = Y22;
Y66 = -Y13;
Y67 = 0;
Y68 = t5 - t11;
Y69 = Y24;
Y610 = -Y14;
Y611 = -t7;
Y612 = t7;
Y613 = dwz;

YB52 = [Y11 Y12 Y13 Y14 Y15 Y16 Y17 Y18 Y19 Y110 Y111 Y112 Y113;...
        Y21 Y22 Y23 Y24 Y25 Y26 Y27 Y28 Y29 Y210 Y211 Y212 Y213;...
        Y31 Y32 Y33 Y34 Y35 Y36 Y37 Y38 Y39 Y310 Y311 Y312 Y313;...
        Y41 Y42 Y43 Y44 Y45 Y46 Y47 Y48 Y49 Y410 Y411 Y412 Y413;...
        Y51 Y52 Y53 Y54 Y55 Y56 Y57 Y58 Y59 Y510 Y511 Y512 Y513;...
        Y61 Y62 Y63 Y64 Y65 Y66 Y67 Y68 Y69 Y610 Y611 Y612 Y613];

== matlab function SimForcesGP2020a/Hydraulic manipulator, calculation/AnalyticTotalForces/Structure 2 (Prismatic segment)/MATLAB Function3 ==
  data: thetaP32 output; P32_r_P32C parameter; mP32 parameter; P32cI parameter
function thetaP32 = thetaP32(P32_r_P32C, mP32, P32cI)

rx = P32_r_P32C(1);
ry = P32_r_P32C(2);
rz = P32_r_P32C(3);

Ixx = P32cI(1,1);
Iyy = P32cI(2,2);
Izz = P32cI(3,3);
Iyz = P32cI(2,3);
Ixz = P32cI(1,3);
Ixy = P32cI(1,2);

t1 = rx*rx;
t2 = ry*ry;
t3 = rz*rz;
t4 = rx*mP32;

thetaP32 = [mP32; rx*mP32; ry*mP32; rz*mP32; t1*mP32; t2*mP32; t3*mP32; t4*ry - Ixy; t4*rz - Ixz; mP32*ry*rz - Iyz; Ixx; Iyy; Izz];

== matlab function SimForcesGP2020a/Hydraulic manipulator, calculation/AnalyticVelocities/Structure 2 (Revolute segment)/GeomPropS2R/Subsystem4/q21AngularVelocity ==
  data: x2 input; dx2 input; q21 input; dq21 output; L2 parameter; x20 parameter
function dq21 = dq21(x2, dx2, q21, L2, x20)

dq21 = -((x2+x20)-L2*cos(q21))/((x2+x20)*L2*sin(q21))*dx2;

== matlab function SimForcesGP2020a/Hydraulic manipulator, calculation/AnalyticVelocities/Structure 2 (Revolute segment)/GeomPropS2R/Subsystem5/q22AngularVelocity ==
  data: x2 input; dx2 input; q22 input; dq22 output; L21 parameter; x20 parameter
function dq22 = dq22(x2, dx2, q22, L21, x20)

dq22 = -((x2+x20)-L21*cos(q22))/((x2+x20)*L21*sin(q22))*dx2;

== matlab function SimForcesGP2020a/Hydraulic manipulator, calculation/AnalyticVelocities/Structure 2 (Revolute segment)/GeomPropS2R/TiltPistonVelocity/TiltPistonVelocity ==
  data: x2 input; q2 input; dq2 input; dx2 output; L2 parameter; L21 parameter; x20 parameter
function dx2 = dx2(x2, q2, dq2, L2, L21, x20)

dx2 = -(L2*L21*sin(q2))/(x2+x20)*dq2;

== matlab function SimForcesGP2020a/Hydraulic manipulator, calculation/AnalyticTotalForces/Structure 2 (Prismatic segment)/MATLAB Function4 ==
  data: P32V input; P32a input; P32w input; P32dw input; P32_Rot_W input; Wg parameter; YP32 output
function YP32  = thetaP32(P32V, P32a, P32w, P32dw, P32_Rot_W,  Wg)

vx = P32V(1);
vy = P32V(2);
vz = P32V(3);
ax = P32a(1);
ay = P32a(2);
az = P32a(3);
wx = P32w(1);
wy = P32w(2);
wz = P32w(3);
dwx = P32dw(1);
dwy = P32dw(2);
dwz = P32dw(3);
P32g = P32_Rot_W*Wg;
gx = P32g(1);
gy = P32g(2);
gz = P32g(3);

Y11 = ( ax + vz * wy - vy * wz  + gx);
t5 = (wy *  wy);
t6 = (wz * wz);
Y12 = -t5 - t6;
t7 = (wx * wy);
Y13 = (t7 - dwz);
t8 = (wx * wz);
Y14 = (t8 + dwy);
Y15 = 0;
Y16 = 0;
Y17 = 0;
Y18 = 0;
Y19 = 0;
Y110 = 0;
Y111 = 0;
Y112 = 0;
Y113 = 0;
Y21 = vx * wz - vz * wx + ay + gy;
Y22 = t7 + dwz;
t11 = wx * wx;
Y23 = -t11 - t6;
t12 = wy * wz;
Y24 = t12 - dwx;
Y25 = 0;
Y26 = 0;
Y27 = 0;
Y28 = 0;
Y29 = 0;
Y210 = 0;
Y211 = 0;
Y212 = 0;
Y213 = 0;
Y31 = -vx * wy + vy * wx + az + gz;
Y32 = t8 - dwy;
Y33 = t12 + dwx;
Y34 = -t11 - t5;
Y35 = 0;
Y36 = 0;
Y37 = 0;
Y38 = 0;
Y39 = 0;
Y310 = 0;
Y311 = 0;
Y312 = 0;
Y313 = 0;
Y41 = 0;
Y42 = 0;
Y43 = Y31;
Y44 = -Y21;
Y45 = 0;
Y46 = Y33;
Y47 = -Y24;
Y48 = Y32;
Y49 = -Y22;
Y410 = -t5 + t6;
Y411 = dwx;
Y412 = -t12;
Y413 = t12;
Y51 = 0;
Y52 = -Y31;
Y53 = 0;
Y54 = Y11;
Y55 = -Y32;
Y56 = 0;
Y57 = Y14;
Y58 = -Y33;
Y59 = t11 - t6;
Y510 = Y13;
Y511 = t8;
Y512 = dwy;
Y513 = -t8;
Y61 = 0;
Y62 = Y21;
Y63 = -Y11;
Y64 = 0;
Y65 = Y22;
Y66 = -Y13;
Y67 = 0;
Y68 = t5 - t11;
Y69 = Y24;
Y610 = -Y14;
Y611 = -t7;
Y612 = t7;
Y613 = dwz;

YP32 = [Y11 Y12 Y13 Y14 Y15 Y16 Y17 Y18 Y19 Y110 Y111 Y112 Y113;...
        Y21 Y22 Y23 Y24 Y25 Y26 Y27 Y28 Y29 Y210 Y211 Y212 Y213;...
        Y31 Y32 Y33 Y34 Y35 Y36 Y37 Y38 Y39 Y310 Y311 Y312 Y313;...
        Y41 Y42 Y43 Y44 Y45 Y46 Y47 Y48 Y49 Y410 Y411 Y412 Y413;...
        Y51 Y52 Y53 Y54 Y55 Y56 Y57 Y58 Y59 Y510 Y511 Y512 Y513;...
        Y61 Y62 Y63 Y64 Y65 Y66 Y67 Y68 Y69 Y610 Y611 Y612 Y613];

== matlab function SimForcesGP2020a/Hydraulic manipulator, calculation/AnalyticVelocities/Structure 2 (Prismatic segment)/UMatsS2P/P32_U_D22 ==
  data: P32_r_P32D22 input; P32_U_D22 output; P32_Rot_D22 input
function P32_U_D22 = P32_U_D22(P32_r_P32D22, P32_Rot_D22)

P32_U_D22 = [P32_Rot_D22,                    zeros(3);...
              dual(P32_r_P32D22)*P32_Rot_D22, P32_Rot_D22];
   
end
   
function dual_r = dual(ArAB)

dual_r = [0,  -ArAB(3), ArAB(2);...
          ArAB(3), 0, -ArAB(1);...
          -ArAB(2), ArAB(1), 0];

end

== matlab function SimForcesGP2020a/Hydraulic manipulator, calculation/AnalyticVelocities/Structure 1/GeomPropS1/Subsystem1/q11AngularVelocity ==
  data: x1 input; q11 input; dx1 input; dq11 output; L1 parameter; x10 parameter
function dq11 = dq11(x1, q11, dx1, L1, x10)

dq11 = -((x1+x10)-L1*cos(q11))/((x1+x10)*L1*sin(q11))*dx1;

== matlab function SimForcesGP2020a/Hydraulic manipulator, calculation/AnalyticTotalForces/Structure 1/MATLAB Function ==
  data: thetaBc1 output; Bc1_r_Bc1C parameter; mBc1 parameter; Bc1cI parameter
function thetaBc1 = thetaBc1(Bc1_r_Bc1C, mBc1, Bc1cI)

rx = Bc1_r_Bc1C(1);
ry = Bc1_r_Bc1C(2);
rz = Bc1_r_Bc1C(3);

Ixx = Bc1cI(1,1);
Iyy = Bc1cI(2,2);
Izz = Bc1cI(3,3);
Iyz = Bc1cI(2,3);
Ixz = Bc1cI(1,3);
Ixy = Bc1cI(1,2);

t1 = rx*rx;
t2 = ry*ry;
t3 = rz*rz;
t4 = rx*mBc1;

thetaBc1 = [mBc1; rx*mBc1; ry*mBc1; rz*mBc1; t1*mBc1; t2*mBc1; t3*mBc1; t4*ry - Ixy; t4*rz - Ixz; mBc1*ry*rz - Iyz; Ixx; Iyy; Izz];

== matlab function SimForcesGP2020a/Hydraulic manipulator, calculation/AnalyticTotalForces/Structure 1/MATLAB Function1 ==
  data: Bc1V input; Bc1a input; Bc1w input; Bc1dw input; Bc1_Rot_W input; Wg parameter; YBc1 output
function YBc1  = thetaBc1(Bc1V, Bc1a, Bc1w, Bc1dw, Bc1_Rot_W,  Wg)

vx = Bc1V(1);
vy = Bc1V(2);
vz = Bc1V(3);
ax = Bc1a(1);
ay = Bc1a(2);
az = Bc1a(3);
wx = Bc1w(1);
wy = Bc1w(2);
wz = Bc1w(3);
dwx = Bc1dw(1);
dwy = Bc1dw(2);
dwz = Bc1dw(3);
Bc1g = Bc1_Rot_W*Wg;
gx = Bc1g(1);
gy = Bc1g(2);
gz = Bc1g(3);

Y11 = ( ax + vz * wy - vy * wz  + gx);
t5 = (wy *  wy);
t6 = (wz * wz);
Y12 = -t5 - t6;
t7 = (wx * wy);
Y13 = (t7 - dwz);
t8 = (wx * wz);
Y14 = (t8 + dwy);
Y15 = 0;
Y16 = 0;
Y17 = 0;
Y18 = 0;
Y19 = 0;
Y110 = 0;
Y111 = 0;
Y112 = 0;
Y113 = 0;
Y21 = vx * wz - vz * wx + ay + gy;
Y22 = t7 + dwz;
t11 = wx * wx;
Y23 = -t11 - t6;
t12 = wy * wz;
Y24 = t12 - dwx;
Y25 = 0;
Y26 = 0;
Y27 = 0;
Y28 = 0;
Y29 = 0;
Y210 = 0;
Y211 = 0;
Y212 = 0;
Y213 = 0;
Y31 = -vx * wy + vy * wx + az + gz;
Y32 = t8 - dwy;
Y33 = t12 + dwx;
Y34 = -t11 - t5;
Y35 = 0;
Y36 = 0;
Y37 = 0;
Y38 = 0;
Y39 = 0;
Y310 = 0;
Y311 = 0;
Y312 = 0;
Y313 = 0;
Y41 = 0;
Y42 = 0;
Y43 = Y31;
Y44 = -Y21;
Y45 = 0;
Y46 = Y33;
Y47 = -Y24;
Y48 = Y32;
Y49 = -Y22;
Y410 = -t5 + t6;
Y411 = dwx;
Y412 = -t12;
Y413 = t12;
Y51 = 0;
Y52 = -Y31;
Y53 = 0;
Y54 = Y11;
Y55 = -Y32;
Y56 = 0;
Y57 = Y14;
Y58 = -Y33;
Y59 = t11 - t6;
Y510 = Y13;
Y511 = t8;
Y512 = dwy;
Y513 = -t8;
Y61 = 0;
Y62 = Y21;
Y63 = -Y11;
Y64 = 0;
Y65 = Y22;
Y66 = -Y13;
Y67 = 0;
Y68 = t5 - t11;
Y69 = Y24;
Y610 = -Y14;
Y611 = -t7;
Y612 = t7;
Y613 = dwz;

YBc1 = [Y11 Y12 Y13 Y14 Y15 Y16 Y17 Y18 Y19 Y110 Y111 Y112 Y113;...
        Y21 Y22 Y23 Y24 Y25 Y26 Y27 Y28 Y29 Y210 Y211 Y212 Y213;...
        Y31 Y32 Y33 Y34 Y35 Y36 Y37 Y38 Y39 Y310 Y311 Y312 Y313;...
        Y41 Y42 Y43 Y44 Y45 Y46 Y47 Y48 Y49 Y410 Y411 Y412 Y413;...
        Y51 Y52 Y53 Y54 Y55 Y56 Y57 Y58 Y59 Y510 Y511 Y512 Y513;...
        Y61 Y62 Y63 Y64 Y65 Y66 Y67 Y68 Y69 Y610 Y611 Y612 Y613];

== matlab function SimForcesGP2020a/Hydraulic manipulator, calculation/AnalyticVelocities/Structure 1/GeomPropS1/Subsystem2/q12AngularVelocity ==
  data: x1 input; q12 input; dx1 input; dq12 output; L11 parameter; x10 parameter
function dq12 = dq12(x1, q12, dx1, L11, x10)

dq12 = -((x1+x10)-L11*cos(q12))/((x1+x10)*L11*sin(q12))*dx1;

== matlab function SimForcesGP2020a/Hydraulic manipulator, calculation/AnalyticVelocities/Structure 1/UMatsS1/Bc1_U_B31 ==
  data: Bc1_r_Bc1B31 input; Bc1_U_B31 output; Bc1_Rot_B31 input
function Bc1_U_B31 = Bc1_U_B31(Bc1_r_Bc1B31, Bc1_Rot_B31)

Bc1_U_B31 = [Bc1_Rot_B31,                    zeros(3);...
             dual(Bc1_r_Bc1B31)*Bc1_Rot_B31, Bc1_Rot_B31];
   
end
   
function dual_r = dual(ArAB)

dual_r = [0,  -ArAB(3), ArAB(2);...
          ArAB(3), 0, -ArAB(1);...
          -ArAB(2), ArAB(1), 0];

end

== matlab function SimForcesGP2020a/Hydraulic manipulator, calculation/AnalyticVelocities/Structure 1/RotMatsS1/Bc1_Rot_B31 ==
  data: q11 input; Bc1_Rot_B31 output
function Bc1_Rot_B31 = Bc1_Rot_B31(q11)

Bc1_Rot_B31 = [+cos(q11) -sin(q11) 0;...
               +sin(q11) +cos(q11) 0;...
                   0         0     1];
